simulink model "CruiseControl_Intelligent"  (R2022b)
settings: Solver=FixedStepAuto  StartTime=0.0  StopTime=600.0  FixedStep=0.1  RelTol=1e-3  EnableMultiTasking=on
values from neighbouring files (symbols this model uses):
  J = lqr(A,B,Q,R)    [LQR_script.m]
settings Model: Creator=burl  LastModifiedBy=prajw
settings SolverCC: AlgebraicLoopSolver=TrustRegion
settings DataIOCC: ReturnWorkspaceOutputs=off
settings OptimizationCC: LifeSpan=inf
settings DebuggingCC: UnconnectedInputMsg=warning  UnconnectedOutputMsg=warning  UnconnectedLineMsg=warning  SFUnexpectedBacktrackingDiag=warning  SFNoUnconditionalDefaultTransitionDiag=warning  SFExecutionAtInitializationDiag=none  SFMachineParentedDataDiag=warning  ArithmeticOperatorsInVariantConditions=warning
settings ModelReferenceCC: EnableRefExpFcnMdlSchedulingChecks=on
settings SFSimCC: SimUseLocalCustomCode=off  CustomCodeUndefinedFunction=UseInterfaceOnly
settings RTWCC: RTWUseLocalCustomCode=off
settings CodeAppCC: StateflowObjectComments=on
settings GRTTargetCC: TargetLangStandard=C89/C90 (ANSI)
settings ConfigComp: CovMetricSettings=dw  CovSaveCumulativeToWorkspaceVar=on  CovSaveSingleToWorkspaceVar=on  CovExternalEMLEnable=off

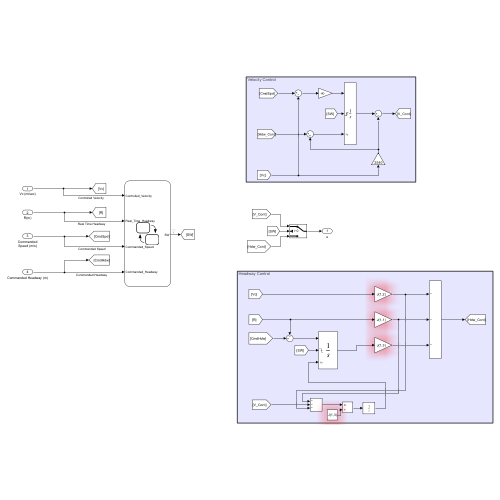
[thumbnail: Simulink's stored preview of the top-level diagram]
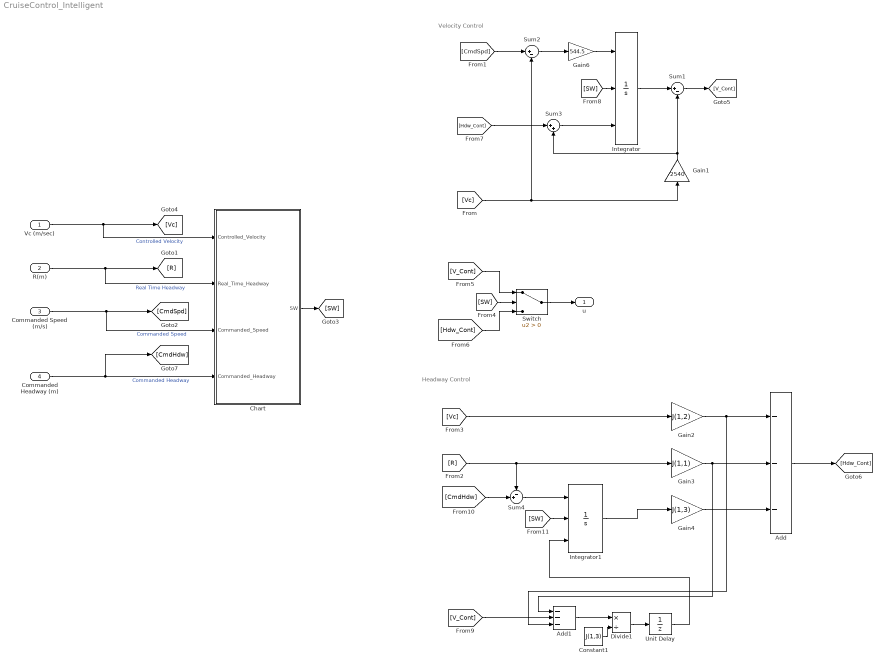
== system CruiseControl_Intelligent ==
  note: Headway Control
  note: Velocity Control
  Vc (m/sec) : Inport
  R(m) : Inport  Port=2
  Commanded Speed (m/s) : Inport  Port=3
  Commanded Headway (m) : Inport  Port=4
  Add : Sum  Inputs=---
  Add1 : Sum  Inputs=---
  Chart : Stateflow chart  TreatAsAtomicUnit=on
  Constant1 : Constant  Value=J(1,3)
  Divide1 : Product  Inputs=*/
  Gain1 : Gain  Gain=2540
  Gain2 : Gain  Gain=J(1,2)
  Gain3 : Gain  Gain=J(1,1)
  Gain4 : Gain  Gain=J(1,3)
  Gain6 : Gain  Gain=544.5
  Integrator : Integrator  ExternalReset=rising  InitialConditionSource=external
  Integrator1 : Integrator  ExternalReset=falling  InitialConditionSource=external
  Sum1 : Sum  Inputs=|+-
  Sum2 : Sum  Inputs=|+-
  Sum3 : Sum  Inputs=|++
  Sum4 : Sum  Inputs=-+|
  Switch : Switch  Criteria=u2 > Threshold  SaturateOnIntegerOverflow=off  InputSameDT=off
  Unit Delay : UnitDelay  SampleTime=-1  HasFrameUpgradeWarning=on
  u : Outport  VectorParamsAs1DForOutWhenUnconnected=off
  wires:
  Switch/1 -> u/1
  [Vc] -> Gain1/1, Sum2/2
  [CmdSpd] -> Sum2/1
  Sum2/1 -> Gain6/1
  Gain1/1 -> Sum1/2, Sum3/2
  Vc (m/sec)/1 -> Chart/1(Controlled_Velocity), [Vc]  "Controlled Velocity"
  Commanded Speed (m/s)/1 -> Chart/3(Commanded_Speed), [CmdSpd]  "Commanded Speed"
  Commanded Headway (m)/1 -> [CmdHdw], Chart/4(Commanded_Headway)  "Commanded Headway"
  Gain4/1 -> Add/3
  Gain3/1 -> Add1/1, Add/2
  [Vc] -> Gain2/1
  Gain2/1 -> Add1/3, Add/1
  Integrator1/1 -> Gain4/1
  R(m)/1 -> [R], Chart/2(Real_Time_Headway)  "Real Time Headway"
  [R] -> Gain3/1, Sum4/1
  Sum1/1 -> [V_Cont]
  [V_Cont] -> Switch/1
  Add/1 -> [Hdw_Cont]
  [Hdw_Cont] -> Switch/3
  Chart/1(SW) -> [SW]
  [Hdw_Cont] -> Sum3/1
  Sum3/1 -> Integrator/3
  [SW] -> Integrator/2
  [V_Cont] -> Add1/2
  [CmdHdw] -> Sum4/2
  Sum4/1 -> Integrator1/1
  [SW] -> Integrator1/2
  Add1/1 -> Divide1/1
  Divide1/1 -> Unit Delay/1
  Unit Delay/1 -> Integrator1/3
  Constant1/1 -> Divide1/2
  [SW] -> Switch/2
  Gain6/1 -> Integrator/1
  Integrator/1 -> Sum1/1

== stateflow chart CruiseControl_Intelligent/Chart ==
  state velocityControl
    entry:
    SW=1
  state headwayControl
    entry:
    SW=0
  (default) -> velocityControl
  velocityControl -> headwayControl : [Real_Time_Headway <= Commanded_Headway && after (5,sec)]
  headwayControl -> velocityControl : [Controlled_Velocity>Commanded_Speed && Real_Time_Headway>Commanded_Headway&& after(5,sec)]
  data: Controlled_Velocity input; Real_Time_Headway input; Commanded_Speed input; SW output; Commanded_Headway input; R parameter
